simulink model "Geschwindigkeitsregler"  (R2015b)
settings: Solver=FixedStepDiscrete  StartTime=0.0  StopTime=9.0  FixedStep=0.01  RelTol=1e-3
values from neighbouring files (symbols this model uses):
  AB1 = zeros(r+1,1)    [ableitung_durch_zvf.m]
  AB2 = zeros(n,1)    [ableitung_durch_zvf.m]
  AD = AD+F    [zvf_design.m]
  BD = BD*K    [zvf_design.m]
  dt = 0.01    [ableitung_durch_zvf.m]
  n = 3    [ableitung_durch_zvf.m]
  r = 3    [ableitung_durch_zvf.m]
undefined symbols (not defined in the file or in its folder): sigbuilder_block
libraries: arduinolib x17, simulink x12
settings Model: SimulationMode=external  ExtModeTrigDuration=2  Creator=Joern  LastModifiedBy=Joern
settings OptimizationCC: OptimizeModelRefInitCode=on  LifeSpan=1  MaxStackSize=64
settings HardwareCC: ProdBitPerInt=16  ProdBitPerPointer=16  ProdLargestAtomicFloat=None  ProdWordSize=8  ProdHWDeviceType=Atmel->AVR
settings RTWCC: SystemTargetFile=ert.tlc  TemplateMakefile=ert_default_tmf  Description=Embedded Coder  Toolchain=Arduino AVR v1.6.1  BuildConfiguration=Faster Runs
settings CodeAppCC: IgnoreCustomStorageClasses=off
settings ERTTargetCC: GenerateSampleERTMain=on  SupportContinuousTime=on  SupportVariableSizeSignals=on

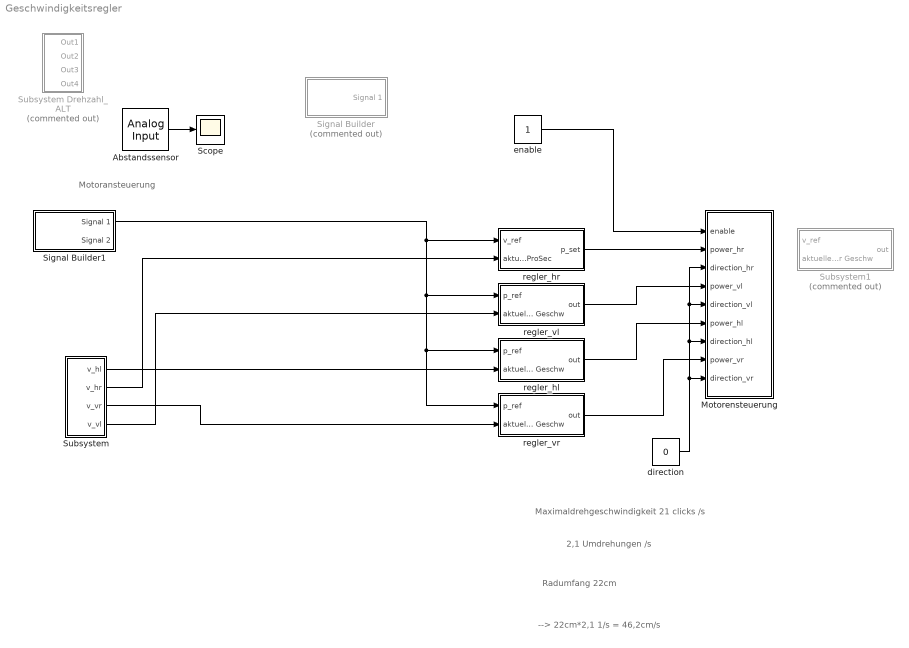
== system Geschwindigkeitsregler ==
  note: --> 22cm*2,1 1/s = 46,2cm/s
  note: Radumfang 22cm
  note: 2,1 Umdrehungen /s
  note: Maximaldrehgeschwindigkeit 21 clicks /s
  note: Motoransteuerung
  Abstandssensor : arduinolib/Analog Input  pinNumber=6  sampleTime=0.1  blockPlatform=arduino
  Motorensteuerung : Subsystem
  Scope : Scope
  Signal Builder : Subsystem  Tag=STV Subsys  Commented=on  LoadFcn=sigbuilder_block('load');  StartFcn=sigbuilder_block('start');  StopFcn=sigbuilder_block('stop');  ClipboardFcn=sigbuilder_block('clipboard');  mask(Sigbuilder block){}
      mask help: Simulink:masks:SigbuilderBlock_MD
      mask init:
      | if ~strcmp(get_param(bdroot(gcbh),'SimulationStatus'),'stopped') tuvar = sigbuilder_block('maskInit'); end
      settings: CopyFcn=sigbuilder_block('copy');  DeleteFcn=sigbuilder_block('delete');  ModelCloseFcn=sigbuilder_block('modelClose');  PreSaveFcn=sigbuilder_block('preSave');  PauseFcn=sigbuilder_block('pause');  ContinueFcn=sigbuilder_block('continue');  NameChangeFcn=sigbuilder_block('namechange');  OpenFcn=sigbuilder_block('open',[6 30 1012.5 447.75 ]);  CloseFcn=sigbuilder_block('close');
      mask Display: plot(0, 0, 100, 100,[2, 2, 32, 32, 2], [68, 8, 8, 68, 68],[32, 2], [38, 38], [32, 19, 2],[53, 60, 44], [32, 17, 17, 2],[16, 16, 31, 31]);txt = getActiveGroup(gcbh);text(2, 100, txt,'verticalAlignment', 'top');
  Signal Builder1 : Subsystem  Tag=STV Subsys  LoadFcn=sigbuilder_block('load');  StartFcn=sigbuilder_block('start');  StopFcn=sigbuilder_block('stop');  ClipboardFcn=sigbuilder_block('clipboard');  mask(Sigbuilder block){}
      mask help: Simulink:masks:SigbuilderBlock_MD
      mask init:
      | if ~strcmp(get_param(bdroot(gcbh),'SimulationStatus'),'stopped') tuvar = sigbuilder_block('maskInit'); end
      settings: CopyFcn=sigbuilder_block('copy');  DeleteFcn=sigbuilder_block('delete');  ModelCloseFcn=sigbuilder_block('modelClose');  PreSaveFcn=sigbuilder_block('preSave');  PauseFcn=sigbuilder_block('pause');  ContinueFcn=sigbuilder_block('continue');  NameChangeFcn=sigbuilder_block('namechange');  OpenFcn=sigbuilder_block('open',[6 30 948 447.75 ]);  CloseFcn=sigbuilder_block('close');
      mask Display: plot(0, 0, 100, 100,[2, 2, 32, 32, 2], [68, 8, 8, 68, 68],[32, 2], [38, 38], [32, 19, 2],[53, 60, 44], [32, 17, 17, 2],[16, 16, 31, 31]);txt = getActiveGroup(gcbh);text(2, 100, txt,'verticalAlignment', 'top');
  Subsystem : Subsystem
  Subsystem Drehzahl_ALT : Subsystem  Commented=on
  Subsystem1 : Subsystem  Commented=on
  direction : Constant  Value=0
  enable : Constant
  regler_hl : Subsystem
  regler_hr : Subsystem
  regler_vl : Subsystem
  regler_vr : Subsystem
  wires:
  enable/1 -> Motorensteuerung/1(enable)
  direction/1 -> Motorensteuerung/9(direction_vr), Motorensteuerung/7(direction_hl), Motorensteuerung/3(direction_hr), Motorensteuerung/5(direction_vl)
  Subsystem/1("v_hl ") -> regler_hl/2("aktuelle umdr Geschw ")
  Subsystem/2("v_hr ") -> regler_hr/2("aktuelle umdr Geschw in clicksProSec ")
  Subsystem/4(v_vl) -> regler_vl/2("aktuelle umdr Geschw ")
  regler_hr/1(p_set) -> Motorensteuerung/2(power_hr)
  Signal Builder1/1(Signal 1) -> regler_hr/1(v_ref), regler_vr/1(p_ref), regler_hl/1(p_ref), regler_vl/1(p_ref)
  regler_vl/1(out) -> Motorensteuerung/4(power_vl)
  regler_hl/1(out) -> Motorensteuerung/6(power_hl)
  regler_vr/1(out) -> Motorensteuerung/8(power_vr)
  Subsystem/3(v_vr) -> regler_vr/2("aktuelle umdr Geschw ")
  Abstandssensor/1 -> Scope/1

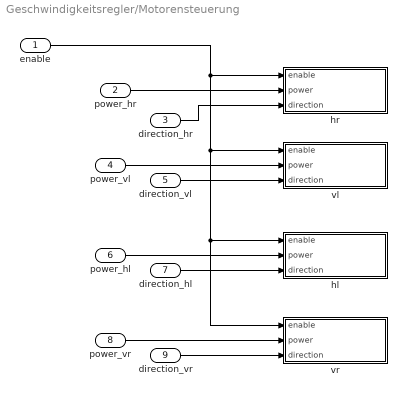
== system Geschwindigkeitsregler/Motorensteuerung ==
  enable : Inport
  power_hr : Inport  Port=2
  direction_hr : Inport  Port=3
  power_vl : Inport  Port=4
  direction_vl : Inport  Port=5
  power_hl : Inport  Port=6
  direction_hl : Inport  Port=7
  power_vr : Inport  Port=8
  direction_vr : Inport  Port=9
  hl : Subsystem  TreatAsAtomicUnit=on
  hr : Subsystem  TreatAsAtomicUnit=on
  vl : Subsystem  TreatAsAtomicUnit=on
  vr : Subsystem  TreatAsAtomicUnit=on
  wires:
  power_vl/1 -> vl/2(power)
  power_hr/1 -> hr/2(power)
  enable/1 -> vr/1(enable), hl/1(enable), vl/1(enable), hr/1(enable)
  direction_hr/1 -> hr/3(direction)
  direction_vl/1 -> vl/3(direction)
  direction_vr/1 -> vr/3(direction)
  power_vr/1 -> vr/2(power)
  direction_hl/1 -> hl/3(direction)
  power_hl/1 -> hl/2(power)

== system Geschwindigkeitsregler/Signal Builder ==
  Demux : Demux  Tag=STV Demux  Outputs=1
  FromWs : FromWorkspace  Tag=STV FromWs  VariableName=tuvar  SampleTime=0
      SigBuilderData=|
      | common.afterFinalStr = 'Extrapolate'
      | common.sampleTime = 0
      | dataSet.timeRange = [0 7]
      | dataSet.name = 'Group 1'
      | sbobj.Groups.Name = 'Group 1'
      | sbobj.Groups.Signals.Name = 'Signal 1'
      | sbobj.Groups.Signals.XData = [0 1 2 4 6 7]
      | sbobj.Groups.Signals.YData = [0 128 128 255 255 0]
      | sbobj.Groups.TimeRange = [0 7]
  Signal 1 : Outport  Tag=STV Outport
  wires:
  FromWs/1 -> Demux/1
  Demux/1 -> Signal 1/1

== system Geschwindigkeitsregler/Signal Builder1 ==
  Demux : Demux  Tag=STV Demux  Outputs=2
  FromWs : FromWorkspace  Tag=STV FromWs  VariableName=tuvar  SampleTime=0  OutputAfterFinalValue=Setting to zero
      SigBuilderData=|
      | common.afterFinalStr = 'Set to zero'
      | common.sampleTime = '0'
      | dataSet.timeRange = [0 7]
      | dataSet.name = 'Group 1'
      | sbobj.Groups.Name = 'Group 1'
      | sbobj.Groups.Signals(1).Name = 'Signal 1'
      | sbobj.Groups.Signals(1).XData = [0 1 2 2 4 6 6 7]
      | sbobj.Groups.Signals(1).YData = [0 0 50 49 49 100 98.5 0]
      | sbobj.Groups.Signals(2).Name = 'Signal 2'
      | sbobj.Groups.Signals(2).XData = [0 7]
      | sbobj.Groups.Signals(2).YData = [100 100]
      | sbobj.Groups.TimeRange = [0 7]
  Signal 1 : Outport  Tag=STV Outport
  Signal 2 : Outport  Tag=STV Outport  Port=2
  wires:
  Demux/1 -> Signal 1/1
  FromWs/1 -> Demux/1
  Demux/2 -> Signal 2/1

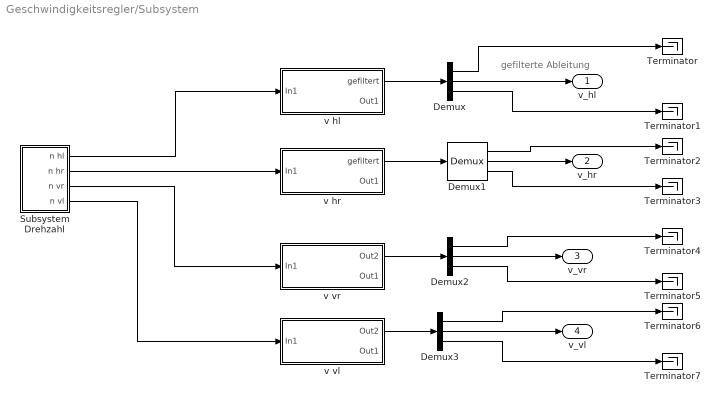
== system Geschwindigkeitsregler/Subsystem ==
  note: gefilterte Ableitung
  Demux{,1..3} (4 alike) : Demux  Outputs=3
  Subsystem Drehzahl : Subsystem
  Terminator{,1..7} (8 alike) : Terminator
  v hl : Subsystem
  v hr : Subsystem
  v vl : Subsystem
  v vr : Subsystem
  "v_hl " : Outport
  "v_hr " : Outport  Port=2
  v_vr : Outport  Port=3
  v_vl : Outport  Port=4
  wires:
  Demux3/2 -> v_vl/1
  v vl/1(Out2) -> Demux3/1
  Demux/2 -> "v_hl "/1
  v vr/1(Out2) -> Demux2/1
  v hr/1(gefiltert) -> Demux1/1
  Demux2/2 -> v_vr/1
  v hl/1(gefiltert) -> Demux/1
  Demux1/2 -> "v_hr "/1
  Subsystem Drehzahl/1(n hl) -> v hl/1(In1)
  Subsystem Drehzahl/2(n hr) -> v hr/1(In1)
  Subsystem Drehzahl/3(n vr) -> v vr/1(In1)
  Subsystem Drehzahl/4(n vl) -> v vl/1(In1)
  Demux/1 -> Terminator/1
  Demux/3 -> Terminator1/1
  Demux1/1 -> Terminator2/1
  Demux1/3 -> Terminator3/1
  Demux2/1 -> Terminator4/1
  Demux2/3 -> Terminator5/1
  Demux3/1 -> Terminator6/1
  Demux3/3 -> Terminator7/1

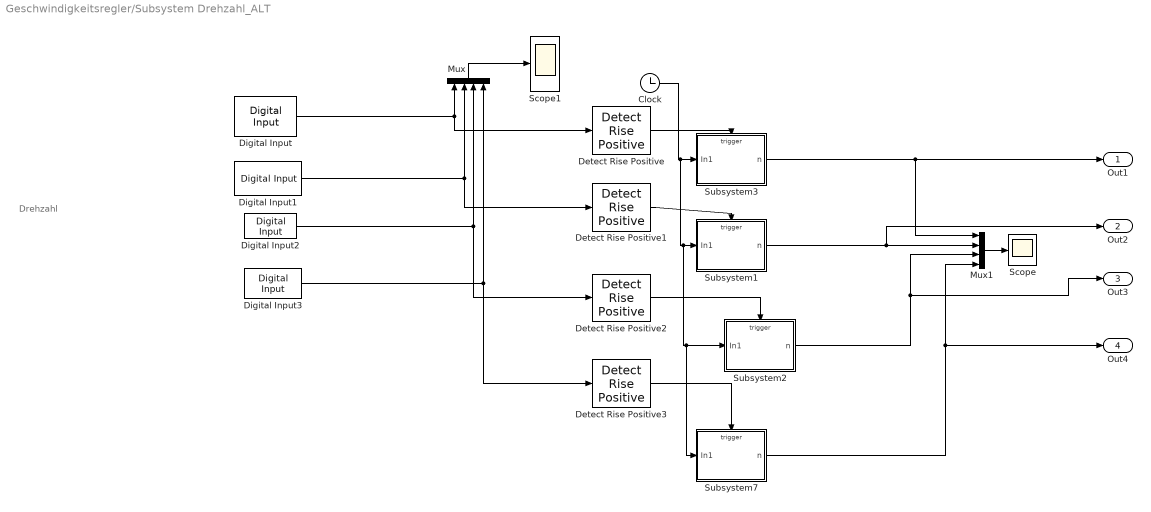
== system Geschwindigkeitsregler/Subsystem Drehzahl_ALT ==
  note: Drehzahl
  Clock : Clock
  Detect Rise Positive{,1..3} (4 alike) : simulink/Logic and Bit Operations/Detect Rise Positive  vinit=0  InputProcessing=Inherited  OutDataTypeStr=boolean
  Digital Input : arduinolib/Digital Input  pinNumber=18  sampleTime=0.01  blockPlatform=arduino
  Digital Input1 : arduinolib/Digital Input  pinNumber=19  sampleTime=0.01  blockPlatform=arduino
  Digital Input2 : arduinolib/Digital Input  pinNumber=2  sampleTime=0.01  blockPlatform=arduino
  Digital Input3 : arduinolib/Digital Input  pinNumber=3  sampleTime=0.01  blockPlatform=arduino
  Mux : Mux
  Mux1 : Mux
  Scope : Scope
  Scope1 : Scope
  Subsystem1 : Subsystem
  Subsystem2 : Subsystem
  Subsystem3 : Subsystem
  Subsystem7 : Subsystem
  Out1 : Outport
  Out2 : Outport  Port=2
  Out3 : Outport  Port=3
  Out4 : Outport  Port=4
  wires:
  Detect Rise Positive1/1 -> Subsystem1/Trigger
  Clock/1 -> Subsystem3/1(In1), Subsystem1/1(In1), Subsystem2/1(In1), Subsystem7/1(In1)
  Detect Rise Positive/1 -> Subsystem3/Trigger
  Digital Input3/1 -> Detect Rise Positive3/1, Mux/4
  Mux1/1 -> Scope/1
  Subsystem2/1(n) -> Mux1/3, Out3/1
  Subsystem3/1(n) -> Mux1/1, Out1/1
  Detect Rise Positive3/1 -> Subsystem7/Trigger
  Detect Rise Positive2/1 -> Subsystem2/Trigger
  Subsystem7/1(n) -> Mux1/4, Out4/1
  Subsystem1/1(n) -> Mux1/2, Out2/1
  Digital Input/1 -> Mux/1, Detect Rise Positive/1
  Digital Input2/1 -> Detect Rise Positive2/1, Mux/3
  Mux/1 -> Scope1/1
  Digital Input1/1 -> Detect Rise Positive1/1, Mux/2

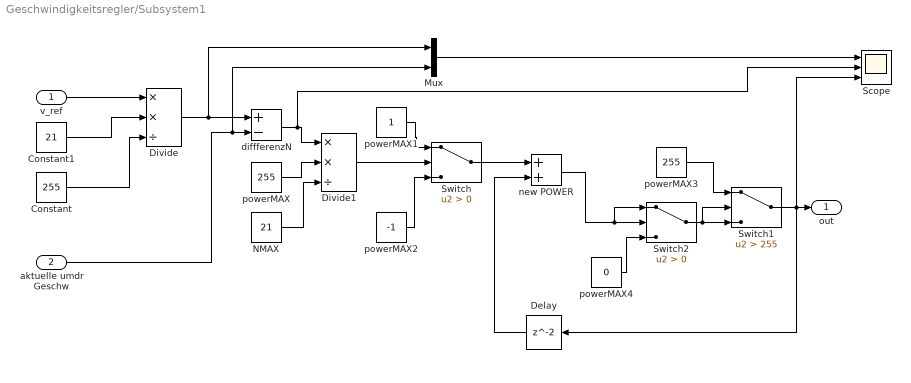
== system Geschwindigkeitsregler/Subsystem1 ==
  v_ref : Inport
  "aktuelle umdr Geschw " : Inport  Port=2
  Constant : Constant  Value=255
  Constant1 : Constant  Value=21
  Delay : Delay
  Divide : Product  Inputs=**/  OutDataTypeStr=double
  Divide1 : Product  Inputs=**/
  Mux : Mux  Inputs=2
  NMAX : Constant  Value=21
  Scope : Scope  NumInputPorts=3
  Switch : Switch  Criteria=u2 > Threshold
  Switch1 : Switch  Criteria=u2 > Threshold  Threshold=255
  Switch2 : Switch  Criteria=u2 > Threshold
  diffferenzN : Sum  Inputs=+-  OutDataTypeStr=double
  new POWER : Sum
  powerMAX : Constant  Value=255
  powerMAX1 : Constant
  powerMAX2 : Constant  Value=-1
  powerMAX3 : Constant  Value=255
  powerMAX4 : Constant  Value=0
  out : Outport
  wires:
  v_ref/1 -> Divide/1
  Constant1/1 -> Divide/2
  Constant/1 -> Divide/3
  Divide/1 -> Mux/1, diffferenzN/1
  "aktuelle umdr Geschw "/1 -> Mux/2, diffferenzN/2
  powerMAX/1 -> Divide1/2
  diffferenzN/1 -> Scope/2, Divide1/1
  NMAX/1 -> Divide1/3
  Delay/1 -> new POWER/2
  powerMAX1/1 -> Switch/1
  powerMAX2/1 -> Switch/3
  Mux/1 -> Scope/1
  Switch2/1 -> Switch1/2, Switch1/3
  Switch1/1 -> Scope/3, Delay/1, out/1
  powerMAX3/1 -> Switch1/1
  powerMAX4/1 -> Switch2/3
  new POWER/1 -> Switch2/1, Switch2/2
  Divide1/1 -> Switch/2
  Switch/1 -> new POWER/1

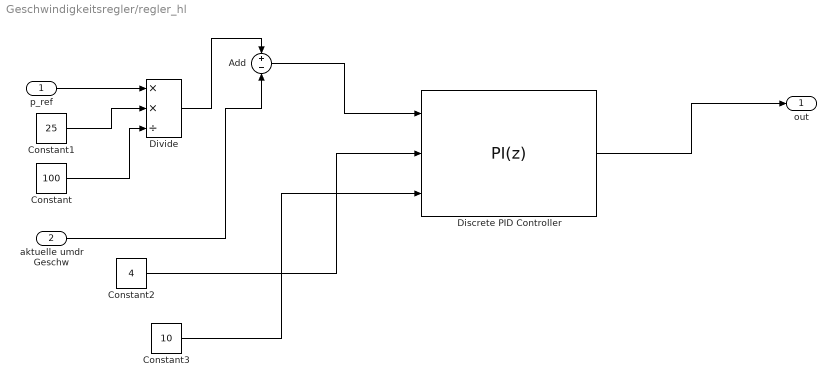
== system Geschwindigkeitsregler/regler_hl ==
  p_ref : Inport
  "aktuelle umdr Geschw " : Inport  Port=2
  Add : Sum  Inputs=+-
  Constant : Constant  Value=100
  Constant1 : Constant  Value=25
  Constant2 : Constant  Value=4
  Constant3 : Constant  Value=10
  Discrete PID Controller : simulink/Continuous/PID Controller  Controller=PI  TimeDomain=Discrete-time  SampleTime=-1  IntegratorMethod=Backward Euler  FilterMethod=Forward Euler  Form=Parallel  UseFilter=on  ControllerParametersSource=external  P=1  I=1  D=0  N=100  InitialConditionSource=internal  InitialConditionForIntegrator=0  InitialConditionForFilter=0  ExternalReset=none  LimitOutput=on  UpperSaturationLimit=255  LowerSaturationLimit=0  LinearizeAsGain=off  AntiWindupMode=none  Kb=1  TrackingMode=off  Kt=1  PParamMin=[]  PParamMax=[]  IParamMin=[]  IParamMax=[]  DParamMin=[]  DParamMax=[]  NParamMin=[]  NParamMax=[]  KbParamMin=[]  KbParamMax=[]  KtParamMin=[]  KtParamMax=[]  POutMin=[]  POutMax=[]  IOutMin=[]  IOutMax=[]  DOutMin=[]  DOutMax=[]  NOutMin=[]  NOutMax=[]  KbOutMin=[]  KbOutMax=[]  KtOutMin=[]  KtOutMax=[]  IntegratorOutMin=[]  IntegratorOutMax=[]  FilterOutMin=[]  FilterOutMax=[]  SumOutMin=[]  SumOutMax=[]  SumI1OutMin=[]  SumI1OutMax=[]  SumI2OutMin=[]  SumI2OutMax=[]  SumI3OutMin=[]  SumI3OutMax=[]  SumDOutMin=[]  SumDOutMax=[]  SaturationOutMin=[]  SaturationOutMax=[]  IntegratorContinuousStateAttributes=''  IntegratorStateMustResolveToSignalObject=off  IntegratorRTWStateStorageClass=Auto  FilterContinuousStateAttributes=''  FilterStateMustResolveToSignalObject=off  FilterRTWStateStorageClass=Auto  DifferentiatorICPrevScaledInput=0  DifferentiatorOutMin=[]  DifferentiatorOutMax=[]
  Divide : Product  Inputs=**/  OutDataTypeStr=double
  out : Outport
  wires:
  Constant/1 -> Divide/3
  Constant1/1 -> Divide/2
  p_ref/1 -> Divide/1
  Divide/1 -> Add/1
  "aktuelle umdr Geschw "/1 -> Add/2
  Add/1 -> Discrete PID Controller/1
  Discrete PID Controller/1 -> out/1
  Constant2/1 -> Discrete PID Controller/2
  Constant3/1 -> Discrete PID Controller/3

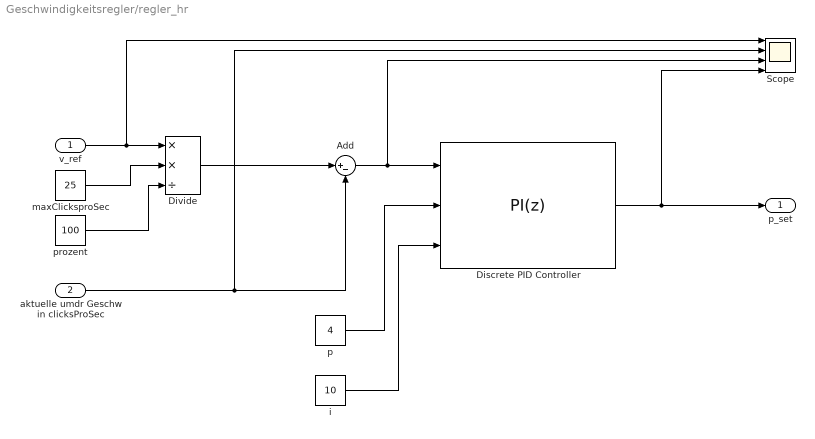
== system Geschwindigkeitsregler/regler_hr ==
  v_ref : Inport
  "aktuelle umdr Geschw in clicksProSec " : Inport  Port=2
  Add : Sum  Inputs=|+-
  Discrete PID Controller : simulink/Continuous/PID Controller  Controller=PI  TimeDomain=Discrete-time  SampleTime=-1  IntegratorMethod=Backward Euler  FilterMethod=Forward Euler  Form=Parallel  UseFilter=on  ControllerParametersSource=external  P=1  I=1  D=0  N=100  InitialConditionSource=internal  InitialConditionForIntegrator=0  InitialConditionForFilter=0  ExternalReset=none  LimitOutput=on  UpperSaturationLimit=255  LowerSaturationLimit=0  LinearizeAsGain=off  AntiWindupMode=none  Kb=1  TrackingMode=off  Kt=1  PParamMin=[]  PParamMax=[]  IParamMin=[]  IParamMax=[]  DParamMin=[]  DParamMax=[]  NParamMin=[]  NParamMax=[]  KbParamMin=[]  KbParamMax=[]  KtParamMin=[]  KtParamMax=[]  POutMin=[]  POutMax=[]  IOutMin=[]  IOutMax=[]  DOutMin=[]  DOutMax=[]  NOutMin=[]  NOutMax=[]  KbOutMin=[]  KbOutMax=[]  KtOutMin=[]  KtOutMax=[]  IntegratorOutMin=[]  IntegratorOutMax=[]  FilterOutMin=[]  FilterOutMax=[]  SumOutMin=[]  SumOutMax=[]  SumI1OutMin=[]  SumI1OutMax=[]  SumI2OutMin=[]  SumI2OutMax=[]  SumI3OutMin=[]  SumI3OutMax=[]  SumDOutMin=[]  SumDOutMax=[]  SaturationOutMin=[]  SaturationOutMax=[]  IntegratorContinuousStateAttributes=''  IntegratorStateMustResolveToSignalObject=off  IntegratorRTWStateStorageClass=Auto  FilterContinuousStateAttributes=''  FilterStateMustResolveToSignalObject=off  FilterRTWStateStorageClass=Auto  DifferentiatorICPrevScaledInput=0  DifferentiatorOutMin=[]  DifferentiatorOutMax=[]
  Divide : Product  Inputs=**/  OutDataTypeStr=double
  Scope : Scope  NumInputPorts=4
  i : Constant  Value=10
  maxClicksproSec : Constant  Value=25
  p : Constant  Value=4
  prozent : Constant  Value=100
  p_set : Outport
  wires:
  prozent/1 -> Divide/3
  maxClicksproSec/1 -> Divide/2
  v_ref/1 -> Scope/1, Divide/1
  Divide/1 -> Add/1
  "aktuelle umdr Geschw in clicksProSec "/1 -> Scope/2, Add/2
  Add/1 -> Scope/3, Discrete PID Controller/1
  Discrete PID Controller/1 -> Scope/4, p_set/1
  p/1 -> Discrete PID Controller/2
  i/1 -> Discrete PID Controller/3

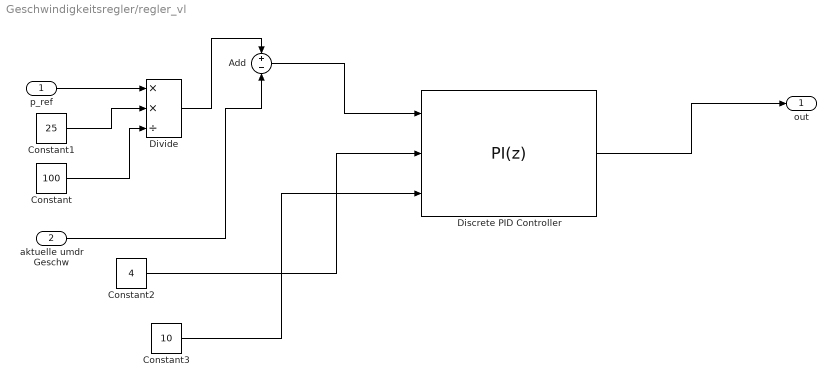
== system Geschwindigkeitsregler/regler_vl ==
  p_ref : Inport
  "aktuelle umdr Geschw " : Inport  Port=2
  Add : Sum  Inputs=+-
  Constant : Constant  Value=100
  Constant1 : Constant  Value=25
  Constant2 : Constant  Value=4
  Constant3 : Constant  Value=10
  Discrete PID Controller : simulink/Continuous/PID Controller  Controller=PI  TimeDomain=Discrete-time  SampleTime=-1  IntegratorMethod=Backward Euler  FilterMethod=Forward Euler  Form=Parallel  UseFilter=on  ControllerParametersSource=external  P=1  I=1  D=0  N=100  InitialConditionSource=internal  InitialConditionForIntegrator=0  InitialConditionForFilter=0  ExternalReset=none  LimitOutput=on  UpperSaturationLimit=255  LowerSaturationLimit=0  LinearizeAsGain=off  AntiWindupMode=none  Kb=1  TrackingMode=off  Kt=1  PParamMin=[]  PParamMax=[]  IParamMin=[]  IParamMax=[]  DParamMin=[]  DParamMax=[]  NParamMin=[]  NParamMax=[]  KbParamMin=[]  KbParamMax=[]  KtParamMin=[]  KtParamMax=[]  POutMin=[]  POutMax=[]  IOutMin=[]  IOutMax=[]  DOutMin=[]  DOutMax=[]  NOutMin=[]  NOutMax=[]  KbOutMin=[]  KbOutMax=[]  KtOutMin=[]  KtOutMax=[]  IntegratorOutMin=[]  IntegratorOutMax=[]  FilterOutMin=[]  FilterOutMax=[]  SumOutMin=[]  SumOutMax=[]  SumI1OutMin=[]  SumI1OutMax=[]  SumI2OutMin=[]  SumI2OutMax=[]  SumI3OutMin=[]  SumI3OutMax=[]  SumDOutMin=[]  SumDOutMax=[]  SaturationOutMin=[]  SaturationOutMax=[]  IntegratorContinuousStateAttributes=''  IntegratorStateMustResolveToSignalObject=off  IntegratorRTWStateStorageClass=Auto  FilterContinuousStateAttributes=''  FilterStateMustResolveToSignalObject=off  FilterRTWStateStorageClass=Auto  DifferentiatorICPrevScaledInput=0  DifferentiatorOutMin=[]  DifferentiatorOutMax=[]
  Divide : Product  Inputs=**/  OutDataTypeStr=double
  out : Outport
  wires:
  Constant3/1 -> Discrete PID Controller/3
  Constant2/1 -> Discrete PID Controller/2
  Discrete PID Controller/1 -> out/1
  Add/1 -> Discrete PID Controller/1
  "aktuelle umdr Geschw "/1 -> Add/2
  Divide/1 -> Add/1
  p_ref/1 -> Divide/1
  Constant1/1 -> Divide/2
  Constant/1 -> Divide/3

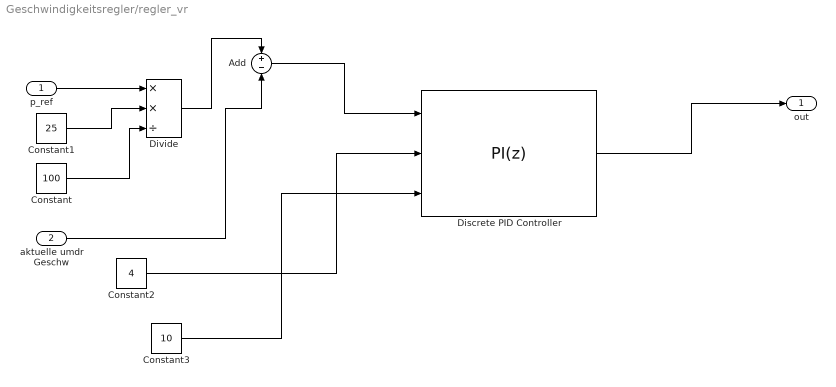
== system Geschwindigkeitsregler/regler_vr ==
  p_ref : Inport
  "aktuelle umdr Geschw " : Inport  Port=2
  Add : Sum  Inputs=+-
  Constant : Constant  Value=100
  Constant1 : Constant  Value=25
  Constant2 : Constant  Value=4
  Constant3 : Constant  Value=10
  Discrete PID Controller : simulink/Continuous/PID Controller  Controller=PI  TimeDomain=Discrete-time  SampleTime=-1  IntegratorMethod=Backward Euler  FilterMethod=Forward Euler  Form=Parallel  UseFilter=on  ControllerParametersSource=external  P=1  I=1  D=0  N=100  InitialConditionSource=internal  InitialConditionForIntegrator=0  InitialConditionForFilter=0  ExternalReset=none  LimitOutput=on  UpperSaturationLimit=255  LowerSaturationLimit=0  LinearizeAsGain=off  AntiWindupMode=none  Kb=1  TrackingMode=off  Kt=1  PParamMin=[]  PParamMax=[]  IParamMin=[]  IParamMax=[]  DParamMin=[]  DParamMax=[]  NParamMin=[]  NParamMax=[]  KbParamMin=[]  KbParamMax=[]  KtParamMin=[]  KtParamMax=[]  POutMin=[]  POutMax=[]  IOutMin=[]  IOutMax=[]  DOutMin=[]  DOutMax=[]  NOutMin=[]  NOutMax=[]  KbOutMin=[]  KbOutMax=[]  KtOutMin=[]  KtOutMax=[]  IntegratorOutMin=[]  IntegratorOutMax=[]  FilterOutMin=[]  FilterOutMax=[]  SumOutMin=[]  SumOutMax=[]  SumI1OutMin=[]  SumI1OutMax=[]  SumI2OutMin=[]  SumI2OutMax=[]  SumI3OutMin=[]  SumI3OutMax=[]  SumDOutMin=[]  SumDOutMax=[]  SaturationOutMin=[]  SaturationOutMax=[]  IntegratorContinuousStateAttributes=''  IntegratorStateMustResolveToSignalObject=off  IntegratorRTWStateStorageClass=Auto  FilterContinuousStateAttributes=''  FilterStateMustResolveToSignalObject=off  FilterRTWStateStorageClass=Auto  DifferentiatorICPrevScaledInput=0  DifferentiatorOutMin=[]  DifferentiatorOutMax=[]
  Divide : Product  Inputs=**/  OutDataTypeStr=double
  out : Outport
  wires:
  Constant3/1 -> Discrete PID Controller/3
  Constant2/1 -> Discrete PID Controller/2
  Discrete PID Controller/1 -> out/1
  Add/1 -> Discrete PID Controller/1
  "aktuelle umdr Geschw "/1 -> Add/2
  Divide/1 -> Add/1
  p_ref/1 -> Divide/1
  Constant1/1 -> Divide/2
  Constant/1 -> Divide/3

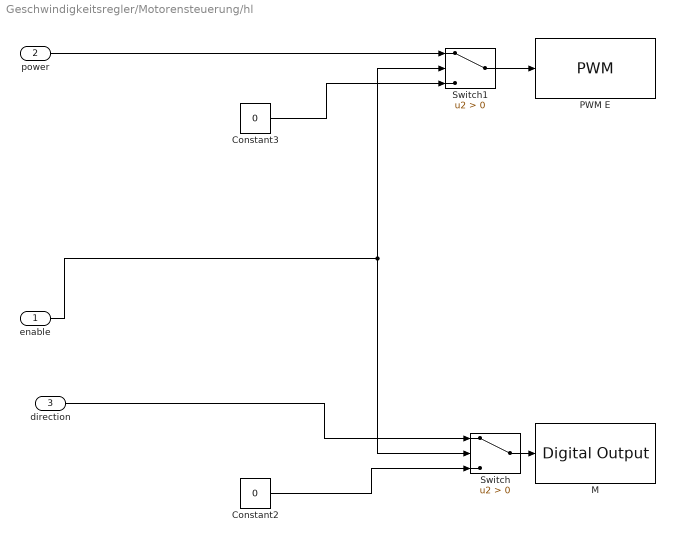
== system Geschwindigkeitsregler/Motorensteuerung/hl ==
  enable : Inport
  power : Inport  Port=2
  direction : Inport  Port=3
  Constant2 : Constant  Value=0
  Constant3 : Constant  Value=0
  M : arduinolib/Digital Output  pinNumber=14  blockPlatform=arduino
  PWM E : arduinolib/PWM  pinNumber=8  blockPlatform=arduino
  Switch : Switch  Criteria=u2 > Threshold
  Switch1 : Switch  Criteria=u2 > Threshold
  wires:
  Switch/1 -> M/1
  Switch1/1 -> PWM E/1
  enable/1 -> Switch/2, Switch1/2
  Constant3/1 -> Switch1/3
  direction/1 -> Switch/1
  Constant2/1 -> Switch/3
  power/1 -> Switch1/1

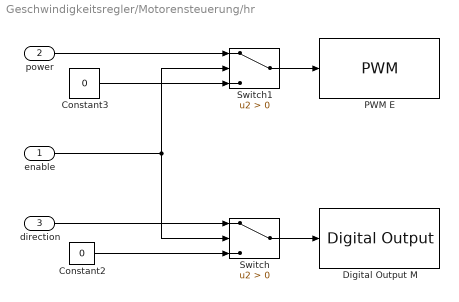
== system Geschwindigkeitsregler/Motorensteuerung/hr ==
  enable : Inport
  power : Inport  Port=2
  direction : Inport  Port=3
  Constant2 : Constant  Value=0
  Constant3 : Constant  Value=0
  Digital Output M : arduinolib/Digital Output  pinNumber=7  blockPlatform=arduino
  PWM E : arduinolib/PWM  pinNumber=6  blockPlatform=arduino
  Switch : Switch  Criteria=u2 > Threshold
  Switch1 : Switch  Criteria=u2 > Threshold
  wires:
  Switch/1 -> Digital Output M/1
  Switch1/1 -> PWM E/1
  enable/1 -> Switch/2, Switch1/2
  Constant3/1 -> Switch1/3
  direction/1 -> Switch/1
  Constant2/1 -> Switch/3
  power/1 -> Switch1/1

== system Geschwindigkeitsregler/Motorensteuerung/vl ==
  enable : Inport
  power : Inport  Port=2
  direction : Inport  Port=3
  Constant2 : Constant  Value=0
  Constant3 : Constant  Value=0
  M : arduinolib/Digital Output  pinNumber=15  blockPlatform=arduino
  PWM E : arduinolib/PWM  pinNumber=9  blockPlatform=arduino
  Switch : Switch  Criteria=u2 > Threshold
  Switch1 : Switch  Criteria=u2 > Threshold
  wires:
  Switch/1 -> M/1
  Switch1/1 -> PWM E/1
  enable/1 -> Switch/2, Switch1/2
  Constant3/1 -> Switch1/3
  direction/1 -> Switch/1
  Constant2/1 -> Switch/3
  power/1 -> Switch1/1

== system Geschwindigkeitsregler/Motorensteuerung/vr ==
  enable : Inport
  power : Inport  Port=2
  direction : Inport  Port=3
  Constant2 : Constant  Value=0
  Constant3 : Constant  Value=0
  Digital Output : arduinolib/Digital Output  pinNumber=4  blockPlatform=arduino
  PWM : arduinolib/PWM  pinNumber=5  blockPlatform=arduino
  Switch : Switch  Criteria=u2 > Threshold
  Switch1 : Switch  Criteria=u2 > Threshold
  wires:
  Switch/1 -> Digital Output/1
  Switch1/1 -> PWM/1
  enable/1 -> Switch/2, Switch1/2
  Constant3/1 -> Switch1/3
  direction/1 -> Switch/1
  Constant2/1 -> Switch/3
  power/1 -> Switch1/1

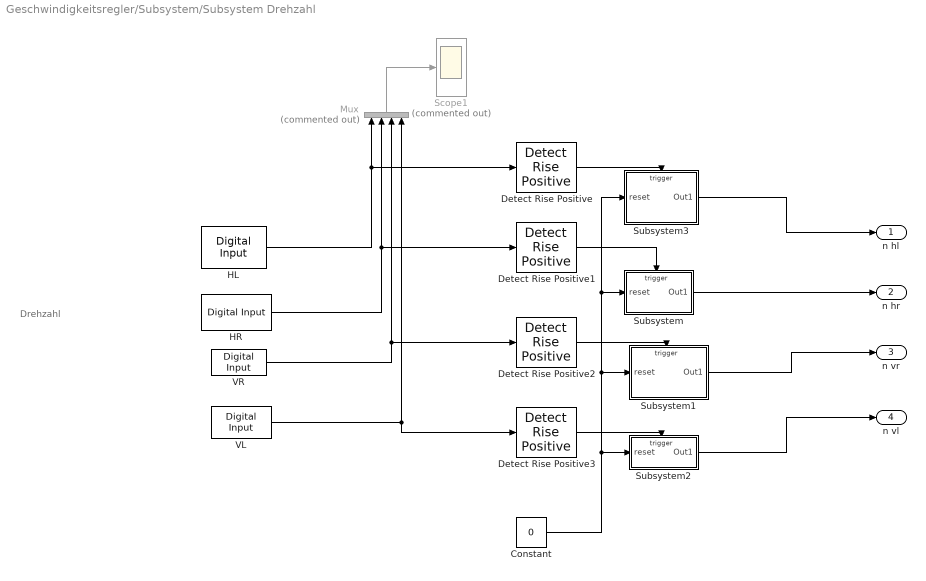
== system Geschwindigkeitsregler/Subsystem/Subsystem Drehzahl ==
  note: Drehzahl
  Constant : Constant  Value=0
  Detect Rise Positive{,1..3} (4 alike) : simulink/Logic and Bit Operations/Detect Rise Positive  vinit=0  InputProcessing=Inherited  OutDataTypeStr=boolean
  HL : arduinolib/Digital Input  pinNumber=18  sampleTime=0.01  blockPlatform=arduino
  HR : arduinolib/Digital Input  pinNumber=19  sampleTime=0.01  blockPlatform=arduino
  Mux : Mux  Commented=on
  Scope1 : Scope  Commented=on
  Subsystem : Subsystem
  Subsystem1 : Subsystem
  Subsystem2 : Subsystem
  Subsystem3 : Subsystem
  VL : arduinolib/Digital Input  pinNumber=3  sampleTime=0.01  blockPlatform=arduino
  VR : arduinolib/Digital Input  pinNumber=2  sampleTime=0.01  blockPlatform=arduino
  n hl : Outport
  n hr : Outport  Port=2
  n vr : Outport  Port=3
  n vl : Outport  Port=4
  wires:
  Mux/1 -> Scope1/1
  HL/1 -> Mux/1, Detect Rise Positive/1
  HR/1 -> Mux/2, Detect Rise Positive1/1
  VR/1 -> Mux/3, Detect Rise Positive2/1
  VL/1 -> Mux/4, Detect Rise Positive3/1
  Detect Rise Positive/1 -> Subsystem3/Trigger
  Detect Rise Positive1/1 -> Subsystem/Trigger
  Detect Rise Positive2/1 -> Subsystem1/Trigger
  Detect Rise Positive3/1 -> Subsystem2/Trigger
  Constant/1 -> Subsystem2/1(reset), Subsystem1/1(reset), Subsystem/1(reset), Subsystem3/1(reset)
  Subsystem3/1(Out1) -> n hl/1
  Subsystem/1(Out1) -> n hr/1
  Subsystem1/1(Out1) -> n vr/1
  Subsystem2/1(Out1) -> n vl/1

== system Geschwindigkeitsregler/Subsystem/v hl ==
  In1 : Inport
  Zustandsvariablenfilter : DiscreteStateSpace  A=AD  B=BD  C=eye(n)  D=zeros(n,r+1)  X0=AB2  SampleTime=dt
  r+1 Altwerte : DiscreteStateSpace  A=[zeros(1,r+1);[eye(r) zeros(r,1)]]  B=[1;zeros(r,1)]  C=eye(r+1)  D=zeros(r+1,1)  X0=AB1  SampleTime=dt
  gefiltert : Outport
  Out1 : Outport  Port=2
  wires:
  In1/1 -> r+1 Altwerte/1
  r+1 Altwerte/1 -> Out1/1, Zustandsvariablenfilter/1
  Zustandsvariablenfilter/1 -> gefiltert/1

== system Geschwindigkeitsregler/Subsystem/v hr ==
  In1 : Inport
  Zustandsvariablenfilter : DiscreteStateSpace  A=AD  B=BD  C=eye(n)  D=zeros(n,r+1)  X0=AB2  SampleTime=dt
  r+1 Altwerte : DiscreteStateSpace  A=[zeros(1,r+1);[eye(r) zeros(r,1)]]  B=[1;zeros(r,1)]  C=eye(r+1)  D=zeros(r+1,1)  X0=AB1  SampleTime=dt
  gefiltert : Outport
  Out1 : Outport  Port=2
  wires:
  Zustandsvariablenfilter/1 -> gefiltert/1
  r+1 Altwerte/1 -> Zustandsvariablenfilter/1, Out1/1
  In1/1 -> r+1 Altwerte/1

== system Geschwindigkeitsregler/Subsystem/v vl ==
  In1 : Inport
  Zustandsvariablenfilter : DiscreteStateSpace  A=AD  B=BD  C=eye(n)  D=zeros(n,r+1)  X0=AB2  SampleTime=dt
  r+1 Altwerte : DiscreteStateSpace  A=[zeros(1,r+1);[eye(r) zeros(r,1)]]  B=[1;zeros(r,1)]  C=eye(r+1)  D=zeros(r+1,1)  X0=AB1  SampleTime=dt
  Out2 : Outport
  Out1 : Outport  Port=2
  wires:
  Zustandsvariablenfilter/1 -> Out2/1
  r+1 Altwerte/1 -> Zustandsvariablenfilter/1, Out1/1
  In1/1 -> r+1 Altwerte/1

== system Geschwindigkeitsregler/Subsystem/v vr ==
  In1 : Inport
  Zustandsvariablenfilter : DiscreteStateSpace  A=AD  B=BD  C=eye(n)  D=zeros(n,r+1)  X0=AB2  SampleTime=dt
  r+1 Altwerte : DiscreteStateSpace  A=[zeros(1,r+1);[eye(r) zeros(r,1)]]  B=[1;zeros(r,1)]  C=eye(r+1)  D=zeros(r+1,1)  X0=AB1  SampleTime=dt
  Out2 : Outport
  Out1 : Outport  Port=2
  wires:
  In1/1 -> r+1 Altwerte/1
  r+1 Altwerte/1 -> Out1/1, Zustandsvariablenfilter/1
  Zustandsvariablenfilter/1 -> Out2/1

== system Geschwindigkeitsregler/Subsystem Drehzahl_ALT/Subsystem1 ==
  In1 : Inport
  Trigger : TriggerPort  PortDimensions=1
  Add1 : Sum  Inputs=+-
  Constant : Constant  Value=1/10
  Delay1 : Delay  DelayLength=1  InitialCondition=0
  Divide : Product  Inputs=*/
  n : Outport
  wires:
  In1/1 -> Add1/1, Delay1/1
  Delay1/1 -> Add1/2
  Add1/1 -> Divide/2
  Constant/1 -> Divide/1
  Divide/1 -> n/1

== system Geschwindigkeitsregler/Subsystem Drehzahl_ALT/Subsystem2 ==
  In1 : Inport
  Trigger : TriggerPort  PortDimensions=1
  Add1 : Sum  Inputs=+-
  Constant : Constant  Value=1/10
  Delay1 : Delay  DelayLength=1  InitialCondition=0
  Divide : Product  Inputs=*/
  n : Outport
  wires:
  Divide/1 -> n/1
  Constant/1 -> Divide/1
  Add1/1 -> Divide/2
  Delay1/1 -> Add1/2
  In1/1 -> Delay1/1, Add1/1

== system Geschwindigkeitsregler/Subsystem Drehzahl_ALT/Subsystem3 ==
  In1 : Inport
  Trigger : TriggerPort  PortDimensions=1
  Add1 : Sum  Inputs=+-
  Constant : Constant  Value=1/10
  Delay1 : Delay  DelayLength=1  InitialCondition=0
  Divide : Product  Inputs=*/
  n : Outport
  wires:
  Divide/1 -> n/1
  Constant/1 -> Divide/1
  Add1/1 -> Divide/2
  Delay1/1 -> Add1/2
  In1/1 -> Delay1/1, Add1/1

== system Geschwindigkeitsregler/Subsystem Drehzahl_ALT/Subsystem7 ==
  In1 : Inport
  Trigger : TriggerPort  PortDimensions=1
  Add1 : Sum  Inputs=+-
  Constant : Constant  Value=1/10
  Delay1 : Delay  DelayLength=1  InitialCondition=0
  Divide : Product  Inputs=*/
  n : Outport
  wires:
  In1/1 -> Add1/1, Delay1/1
  Delay1/1 -> Add1/2
  Add1/1 -> Divide/2
  Constant/1 -> Divide/1
  Divide/1 -> n/1

== system Geschwindigkeitsregler/Subsystem/Subsystem Drehzahl/Subsystem ==
  reset : Inport
  Trigger : TriggerPort  PortDimensions=1
  Add : Sum  Inputs=2
  Constant : Constant
  Constant1 : Constant  Value=0
  Delay : Delay  DelayLength=1  InitialCondition=0
  Switch : Switch  Criteria=u2 > Threshold
  Out1 : Outport
  wires:
  Add/1 -> Delay/1, Out1/1
  Constant/1 -> Add/2
  reset/1 -> Switch/2
  Constant1/1 -> Switch/1
  Switch/1 -> Add/1
  Delay/1 -> Switch/3

== system Geschwindigkeitsregler/Subsystem/Subsystem Drehzahl/Subsystem1 ==
  reset : Inport
  Trigger : TriggerPort  PortDimensions=1
  Add : Sum  Inputs=2
  Constant : Constant
  Constant1 : Constant  Value=0
  Delay : Delay  DelayLength=1  InitialCondition=0
  Switch : Switch  Criteria=u2 > Threshold
  Out1 : Outport
  wires:
  Delay/1 -> Switch/3
  Switch/1 -> Add/1
  Constant1/1 -> Switch/1
  reset/1 -> Switch/2
  Constant/1 -> Add/2
  Add/1 -> Out1/1, Delay/1

== system Geschwindigkeitsregler/Subsystem/Subsystem Drehzahl/Subsystem2 ==
  reset : Inport
  Trigger : TriggerPort  PortDimensions=1
  Add : Sum  Inputs=2
  Constant : Constant
  Constant1 : Constant  Value=0
  Delay : Delay  DelayLength=1  InitialCondition=0
  Switch : Switch  Criteria=u2 > Threshold
  Out1 : Outport
  wires:
  Add/1 -> Delay/1, Out1/1
  Constant/1 -> Add/2
  reset/1 -> Switch/2
  Constant1/1 -> Switch/1
  Switch/1 -> Add/1
  Delay/1 -> Switch/3

== system Geschwindigkeitsregler/Subsystem/Subsystem Drehzahl/Subsystem3 ==
  reset : Inport
  Trigger : TriggerPort  PortDimensions=1
  Add : Sum  Inputs=2
  Constant : Constant
  Constant1 : Constant  Value=0
  Delay : Delay  DelayLength=1  InitialCondition=0
  Switch : Switch  Criteria=u2 > Threshold
  Out1 : Outport
  wires:
  Delay/1 -> Switch/3
  Switch/1 -> Add/1
  Constant1/1 -> Switch/1
  reset/1 -> Switch/2
  Constant/1 -> Add/2
  Add/1 -> Out1/1, Delay/1
